simulink model "Motor_realtime"  (R2024a)
settings: Solver=FixedStepAuto  StartTime=0.0  StopTime=10  FixedStep=MotorSampleTime  RelTol=1e-3
model workspace (MAT data in the model file):
  MotorSampleTime = 0.001
undefined symbols (not defined in the file): Serial_Port, Standard_Devices
libraries: sldrtlib x4
settings Model: Creator=17739  LastModifiedBy=17739

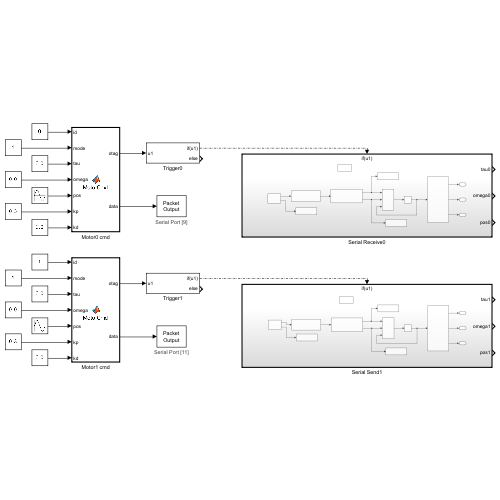
[thumbnail: Simulink's stored preview of the top-level diagram]
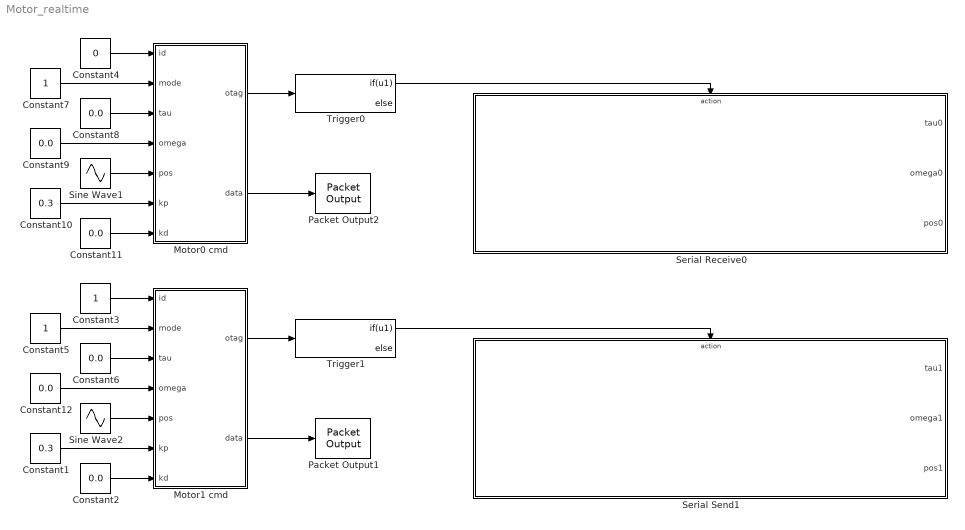
== system Motor_realtime ==
  Constant1 : Constant  Value=0.3
  Constant10 : Constant  Value=0.3
  Constant{2,6,8..9,11..12} (6 alike) : Constant  Value=0.0
  Constant3 : Constant
  Constant4 : Constant  Value=0
  Constant5 : Constant
  Constant7 : Constant
  Motor0 cmd : MATLAB Function  TreatAsAtomicUnit=on
  Motor1 cmd : MATLAB Function  TreatAsAtomicUnit=on
  Packet Output1 : sldrtlib/Packet Output  SampleTime=MotorSampleTime  MaxMissedTicks=inf  ShowMissedTicks=off  YieldWhenWaiting=off  DrvName=Standard_Devices/Serial_Port  DrvAddress=11  DrvOptions=[4000000 8 0 0 0 0 0 0]  PacketSize=17  DataTypes='17*uint8'  ShowReady=off  ShowError=off  PacketID=1  ByteOrder=1  InitialValue=[]  FinalValue=[]
      settings: AttributesFormatString=Serial Port [11]
  Packet Output2 : sldrtlib/Packet Output  SampleTime=MotorSampleTime  MaxMissedTicks=inf  ShowMissedTicks=off  YieldWhenWaiting=off  DrvName=Standard_Devices/Serial_Port  DrvAddress=9  DrvOptions=[4000000 8 0 0 0 0 0 0]  PacketSize=17  DataTypes='17*uint8'  ShowReady=off  ShowError=off  PacketID=1  ByteOrder=1  InitialValue=[]  FinalValue=[]
      settings: AttributesFormatString=Serial Port [9]
  Serial Receive0 : Subsystem  TreatAsAtomicUnit=on
  Serial Send1 : Subsystem  TreatAsAtomicUnit=on
  Sine Wave1 : Sin  Amplitude=pi  Frequency=pi/5  SampleTime=0
  Sine Wave2 : Sin  Amplitude=pi  Frequency=pi/5  SampleTime=0
  Trigger0 : If  IfExpression=u1
  Trigger1 : If  IfExpression=u1
  wires:
  Constant7/1 -> Motor0 cmd/2(mode)
  Constant11/1 -> Motor0 cmd/7(kd)
  Constant4/1 -> Motor0 cmd/1(id)
  Constant8/1 -> Motor0 cmd/3(tau)
  Constant10/1 -> Motor0 cmd/6(kp)
  Constant9/1 -> Motor0 cmd/4(omega)
  Motor0 cmd/2(data) -> Packet Output2/1
  Sine Wave1/1 -> Motor0 cmd/5(pos)
  Sine Wave2/1 -> Motor1 cmd/5(pos)
  Constant3/1 -> Motor1 cmd/1(id)
  Motor1 cmd/2(data) -> Packet Output1/1
  Constant6/1 -> Motor1 cmd/3(tau)
  Constant5/1 -> Motor1 cmd/2(mode)
  Constant1/1 -> Motor1 cmd/6(kp)
  Constant2/1 -> Motor1 cmd/7(kd)
  Constant12/1 -> Motor1 cmd/4(omega)
  Trigger0/1 -> Serial Receive0/Action
  Motor0 cmd/1(otag) -> Trigger0/1
  Trigger1/1 -> Serial Send1/Action
  Motor1 cmd/1(otag) -> Trigger1/1

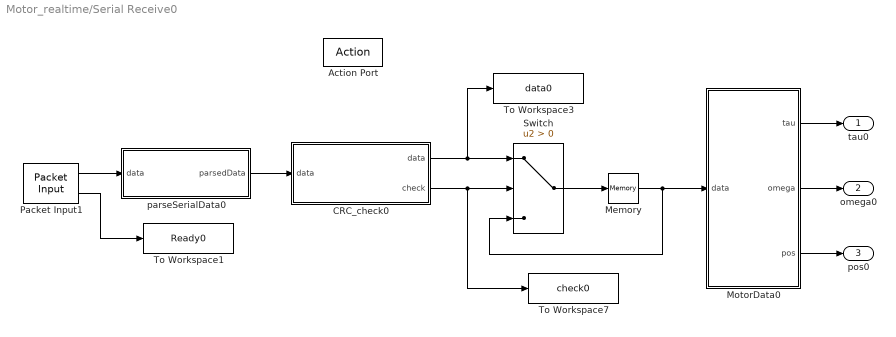
== system Motor_realtime/Serial Receive0 ==
  Action Port : ActionPort  ActionPortLabel=if(u1)
  CRC_check0 : MATLAB Function  TreatAsAtomicUnit=on
  Memory : Memory  InheritSampleTime=on
  MotorData0 : MATLAB Function  TreatAsAtomicUnit=on
  Packet Input1 : sldrtlib/Packet Input  SampleTime=-1  MaxMissedTicks=inf  ShowMissedTicks=off  YieldWhenWaiting=off  DrvName=Standard_Devices/Serial_Port  DrvAddress=9  DrvOptions=[4000000 8 0 0 0 0 0 0]  PacketSize=16  DataTypes='16*uint8'  ShowReady=on  ShowError=off  PacketID=1  ByteOrder=1  ShowTimestamp=off
      settings: AttributesFormatString=Serial Port [9]
  Switch : Switch  Criteria=u2 > Threshold  SaturateOnIntegerOverflow=off  InputSameDT=off
  To Workspace1 : ToWorkspace  VariableName=Ready0  SampleTime=-1
  To Workspace3 : ToWorkspace  VariableName=data0  SampleTime=-1
  To Workspace7 : ToWorkspace  VariableName=check0  SampleTime=-1
  parseSerialData0 : MATLAB Function  TreatAsAtomicUnit=on
  tau0 : Outport
  omega0 : Outport  Port=2
  pos0 : Outport  Port=3
  wires:
  Switch/1 -> Memory/1
  CRC_check0/1(data) -> To Workspace3/1, Switch/1
  CRC_check0/2(check) -> Switch/2, To Workspace7/1
  parseSerialData0/1(parsedData) -> CRC_check0/1("data ")
  Memory/1 -> MotorData0/1(data), Switch/3
  Packet Input1/1 -> parseSerialData0/1(data)
  Packet Input1/2 -> To Workspace1/1
  MotorData0/1(tau) -> tau0/1
  MotorData0/2(omega) -> omega0/1
  MotorData0/3(pos) -> pos0/1

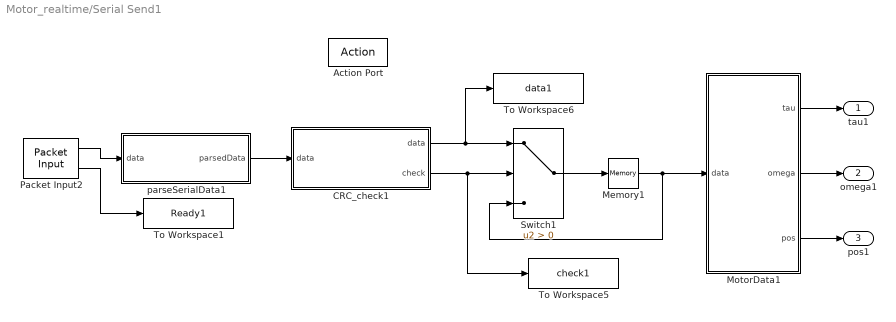
== system Motor_realtime/Serial Send1 ==
  Action Port : ActionPort  ActionPortLabel=if(u1)
  CRC_check1 : MATLAB Function  TreatAsAtomicUnit=on
  Memory1 : Memory  InheritSampleTime=on
  MotorData1 : MATLAB Function  TreatAsAtomicUnit=on
  Packet Input2 : sldrtlib/Packet Input  SampleTime=-1  MaxMissedTicks=inf  ShowMissedTicks=off  YieldWhenWaiting=off  DrvName=Standard_Devices/Serial_Port  DrvAddress=11  DrvOptions=[4000000 8 0 0 0 0 0 0]  PacketSize=16  DataTypes='16*uint8'  ShowReady=on  ShowError=off  PacketID=1  ByteOrder=1  ShowTimestamp=off
      settings: AttributesFormatString=Serial Port [11]
  Switch1 : Switch  Criteria=u2 > Threshold  SaturateOnIntegerOverflow=off  InputSameDT=off
  To Workspace1 : ToWorkspace  VariableName=Ready1  SampleTime=-1
  To Workspace5 : ToWorkspace  VariableName=check1  SampleTime=-1
  To Workspace6 : ToWorkspace  VariableName=data1  SampleTime=-1
  parseSerialData1 : MATLAB Function  TreatAsAtomicUnit=on
  tau1 : Outport
  omega1 : Outport  Port=2
  pos1 : Outport  Port=3
  wires:
  CRC_check1/1(data) -> To Workspace6/1, Switch1/1
  CRC_check1/2(check) -> Switch1/2, To Workspace5/1
  Switch1/1 -> Memory1/1
  Memory1/1 -> MotorData1/1(data), Switch1/3
  parseSerialData1/1(parsedData) -> CRC_check1/1("data ")
  Packet Input2/1 -> parseSerialData1/1(data)
  MotorData1/3(pos) -> pos1/1
  MotorData1/2(omega) -> omega1/1
  MotorData1/1(tau) -> tau1/1
  Packet Input2/2 -> To Workspace1/1

== matlab function Motor_realtime/Serial Send1/parseSerialData1 ==
  data: data input; parsedData output
function parsedData = parseSerialData(data)
    persistent buffer;
    if isempty(buffer)
        buffer = uint8([]);
    end

    % Append new data to buffer, ensuring data is a row vector
    buffer = [buffer, data(:)']; 

    % Define header and data size
    header = uint8([253, 238]); % 定义包头
    dataSize = 16; % 你的数据包大小

    % Initialize parsedData as an empty uint8 array of size 16
    parsedData = uint8([253, 238, zeros(1, dataSize-2)]);

    % Check if the buffer contains a valid packet
    while length(buffer) >= dataSize
        % Find the header in the buffer
        headerPos = findHeader(buffer, header);

        % If header is found and there is enough data for a full packet
        if ~isempty(headerPos) && (headerPos(1) + dataSize - 1 <= length(buffer))
            % Extract the valid packet
            for num = 1:dataSize
                parsedData(num) = buffer(headerPos(1) + num - 1);
            end
            % Remove the extracted packet from the buffer
            if length(headerPos) > 1
                buffer = buffer(headerPos(2):end);
            else
                buffer = buffer((headerPos(1) + dataSize):end);
            end
            return; % Exit the function after finding the first valid packet
        else
            % If no valid packet is found, clear the buffer up to the header position
            if ~isempty(headerPos)
                buffer = buffer(headerPos(1):end);
            else
                buffer = uint8([]);
            end
            break;
        end
    end
end

function pos = findHeader(buffer, header)
    pos = [];
    for i = 1:(length(buffer) - length(header) + 1)
        if all(buffer(i:i + length(header) - 1) == header)
            pos = i;
            return;
        end
    end
end

== matlab function Motor_realtime/Motor0 cmd ==
  data: otag output boolean size=1; data output size=[1 17]; id input; mode input; tau input; omega input; pos input; kp input; kd input
function [otag, data] = MotorCmd(id, mode, tau, omega, pos, kp, kd)
otag = true;
data = uint8([hex2dec('FE'), hex2dec('EE'), ...
    mode*16 + id, ...
    typecast(int16(fix(tau * 256)), 'uint8'), ...
    typecast(int16(fix(omega / (2 * pi) * 256)), 'uint8'), ...
    typecast(int32(fix(pos / (2 * pi) * 32768)), 'uint8'), ...
    typecast(int16(fix(kp * 1280)), 'uint8'), ...
    typecast(int16(fix(kd * 1280)), 'uint8'), ...
    0, 0]); % CRC16 计算稍后添加

% 计算并添加 CRC16 校验
crc = calculateCRC(data(1:15)); % 自定义 CRC 计算函数
data(16:17) = typecast(uint16(crc), 'uint8');
end
% 自定义 CRC 计算函数
function crc = calculateCRC(data)
crc_ccitt_table = [
    0x0000, 0x1189, 0x2312, 0x329b, 0x4624, 0x57ad, 0x6536, 0x74bf, ...
    0x8c48, 0x9dc1, 0xaf5a, 0xbed3, 0xca6c, 0xdbe5, 0xe97e, 0xf8f7, ...
    0x1081, 0x0108, 0x3393, 0x221a, 0x56a5, 0x472c, 0x75b7, 0x643e, ...
    0x9cc9, 0x8d40, 0xbfdb, 0xae52, 0xdaed, 0xcb64, 0xf9ff, 0xe876, ...
    0x2102, 0x308b, 0x0210, 0x1399, 0x6726, 0x76af, 0x4434, 0x55bd, ...
    0xad4a, 0xbcc3, 0x8e58, 0x9fd1, 0xeb6e, 0xfae7, 0xc87c, 0xd9f5, ...
    0x3183, 0x200a, 0x1291, 0x0318, 0x77a7, 0x662e, 0x54b5, 0x453c, ...
    0xbdcb, 0xac42, 0x9ed9, 0x8f50, 0xfbef, 0xea66, 0xd8fd, 0xc974, ...
    0x4204, 0x538d, 0x6116, 0x709f, 0x0420, 0x15a9, 0x2732, 0x36bb, ...
    0xce4c, 0xdfc5, 0xed5e, 0xfcd7, 0x8868, 0x99e1, 0xab7a, 0xbaf3, ...
    0x5285, 0x430c, 0x7197, 0x601e, 0x14a1, 0x0528, 0x37b3, 0x263a, ...
    0xdecd, 0xcf44, 0xfddf, 0xec56, 0x98e9, 0x8960, 0xbbfb, 0xaa72, ...
    0x6306, 0x728f, 0x4014, 0x519d, 0x2522, 0x34ab, 0x0630, 0x17b9, ...
    0xef4e, 0xfec7, 0xcc5c, 0xddd5, 0xa96a, 0xb8e3, 0x8a78, 0x9bf1, ...
    0x7387, 0x620e, 0x5095, 0x411c, 0x35a3, 0x242a, 0x16b1, 0x0738, ...
    0xffcf, 0xee46, 0xdcdd, 0xcd54, 0xb9eb, 0xa862, 0x9af9, 0x8b70, ...
    0x8408, 0x9581, 0xa71a, 0xb693, 0xc22c, 0xd3a5, 0xe13e, 0xf0b7, ...
    0x0840, 0x19c9, 0x2b52, 0x3adb, 0x4e64, 0x5fed, 0x6d76, 0x7cff, ...
    0x9489, 0x8500, 0xb79b, 0xa612, 0xd2ad, 0xc324, 0xf1bf, 0xe036, ...
    0x18c1, 0x0948, 0x3bd3, 0x2a5a, 0x5ee5, 0x4f6c, 0x7df7, 0x6c7e, ...
    0xa50a, 0xb483, 0x8618, 0x9791, 0xe32e, 0xf2a7, 0xc03c, 0xd1b5, ...
    0x2942, 0x38cb, 0x0a50, 0x1bd9, 0x6f66, 0x7eef, 0x4c74, 0x5dfd, ...
    0xb58b, 0xa402, 0x9699, 0x8710, 0xf3af, 0xe226, 0xd0bd, 0xc134, ...
    0x39c3, 0x284a, 0x1ad1, 0x0b58, 0x7fe7, 0x6e6e, 0x5cf5, 0x4d7c, ...
    0xc60c, 0xd785, 0xe51e, 0xf497, 0x8028, 0x91a1, 0xa33a, 0xb2b3, ...
    0x4a44, 0x5bcd, 0x6956, 0x78df, 0x0c60, 0x1de9, 0x2f72, 0x3efb, ...
    0xd68d, 0xc704, 0xf59f, 0xe416, 0x90a9, 0x8120, 0xb3bb, 0xa232, ...
    0x5ac5, 0x4b4c, 0x79d7, 0x685e, 0x1ce1, 0x0d68, 0x3ff3, 0x2e7a, ...
    0xe70e, 0xf687, 0xc41c, 0xd595, 0xa12a, 0xb0a3, 0x8238, 0x93b1, ...
    0x6b46, 0x7acf, 0x4854, 0x59dd, 0x2d62, 0x3ceb, 0x0e70, 0x1ff9, ...
    0xf78f, 0xe606, 0xd49d, 0xc514, 0xb1ab, 0xa022, 0x92b9, 0x8330, ...
    0x7bc7, 0x6a4e, 0x58d5, 0x495c, 0x3de3, 0x2c6a, 0x1ef1, 0x0f78 ...
    ];

crc = uint16(0);
for i = 1:length(data)
    tableIndex = bitand(bitxor(crc, uint16(data(i))), uint16(0xff));
    crc = bitxor(bitshift(crc, -8), crc_ccitt_table(tableIndex + 1));
end
end

== matlab function Motor_realtime/Motor1 cmd ==
  data: otag output size=1; data output size=[1 17]; id input; mode input; tau input; omega input; pos input; kp input; kd input
function [otag, data] = MotorCmd(id, mode, tau, omega, pos, kp, kd)
otag = true;
data = uint8([hex2dec('FE'), hex2dec('EE'), ...
    mode*16 + id, ...
    typecast(int16(fix(tau * 256)), 'uint8'), ...
    typecast(int16(fix(omega / (2 * pi) * 256)), 'uint8'), ...
    typecast(int32(fix(pos / (2 * pi) * 32768)), 'uint8'), ...
    typecast(int16(fix(kp * 1280)), 'uint8'), ...
    typecast(int16(fix(kd * 1280)), 'uint8'), ...
    0, 0]); % CRC16 计算稍后添加

% 计算并添加 CRC16 校验
crc = calculateCRC(data(1:15)); % 自定义 CRC 计算函数
data(16:17) = typecast(uint16(crc), 'uint8');
end
% 自定义 CRC 计算函数
function crc = calculateCRC(data)
crc_ccitt_table = [
    0x0000, 0x1189, 0x2312, 0x329b, 0x4624, 0x57ad, 0x6536, 0x74bf, ...
    0x8c48, 0x9dc1, 0xaf5a, 0xbed3, 0xca6c, 0xdbe5, 0xe97e, 0xf8f7, ...
    0x1081, 0x0108, 0x3393, 0x221a, 0x56a5, 0x472c, 0x75b7, 0x643e, ...
    0x9cc9, 0x8d40, 0xbfdb, 0xae52, 0xdaed, 0xcb64, 0xf9ff, 0xe876, ...
    0x2102, 0x308b, 0x0210, 0x1399, 0x6726, 0x76af, 0x4434, 0x55bd, ...
    0xad4a, 0xbcc3, 0x8e58, 0x9fd1, 0xeb6e, 0xfae7, 0xc87c, 0xd9f5, ...
    0x3183, 0x200a, 0x1291, 0x0318, 0x77a7, 0x662e, 0x54b5, 0x453c, ...
    0xbdcb, 0xac42, 0x9ed9, 0x8f50, 0xfbef, 0xea66, 0xd8fd, 0xc974, ...
    0x4204, 0x538d, 0x6116, 0x709f, 0x0420, 0x15a9, 0x2732, 0x36bb, ...
    0xce4c, 0xdfc5, 0xed5e, 0xfcd7, 0x8868, 0x99e1, 0xab7a, 0xbaf3, ...
    0x5285, 0x430c, 0x7197, 0x601e, 0x14a1, 0x0528, 0x37b3, 0x263a, ...
    0xdecd, 0xcf44, 0xfddf, 0xec56, 0x98e9, 0x8960, 0xbbfb, 0xaa72, ...
    0x6306, 0x728f, 0x4014, 0x519d, 0x2522, 0x34ab, 0x0630, 0x17b9, ...
    0xef4e, 0xfec7, 0xcc5c, 0xddd5, 0xa96a, 0xb8e3, 0x8a78, 0x9bf1, ...
    0x7387, 0x620e, 0x5095, 0x411c, 0x35a3, 0x242a, 0x16b1, 0x0738, ...
    0xffcf, 0xee46, 0xdcdd, 0xcd54, 0xb9eb, 0xa862, 0x9af9, 0x8b70, ...
    0x8408, 0x9581, 0xa71a, 0xb693, 0xc22c, 0xd3a5, 0xe13e, 0xf0b7, ...
    0x0840, 0x19c9, 0x2b52, 0x3adb, 0x4e64, 0x5fed, 0x6d76, 0x7cff, ...
    0x9489, 0x8500, 0xb79b, 0xa612, 0xd2ad, 0xc324, 0xf1bf, 0xe036, ...
    0x18c1, 0x0948, 0x3bd3, 0x2a5a, 0x5ee5, 0x4f6c, 0x7df7, 0x6c7e, ...
    0xa50a, 0xb483, 0x8618, 0x9791, 0xe32e, 0xf2a7, 0xc03c, 0xd1b5, ...
    0x2942, 0x38cb, 0x0a50, 0x1bd9, 0x6f66, 0x7eef, 0x4c74, 0x5dfd, ...
    0xb58b, 0xa402, 0x9699, 0x8710, 0xf3af, 0xe226, 0xd0bd, 0xc134, ...
    0x39c3, 0x284a, 0x1ad1, 0x0b58, 0x7fe7, 0x6e6e, 0x5cf5, 0x4d7c, ...
    0xc60c, 0xd785, 0xe51e, 0xf497, 0x8028, 0x91a1, 0xa33a, 0xb2b3, ...
    0x4a44, 0x5bcd, 0x6956, 0x78df, 0x0c60, 0x1de9, 0x2f72, 0x3efb, ...
    0xd68d, 0xc704, 0xf59f, 0xe416, 0x90a9, 0x8120, 0xb3bb, 0xa232, ...
    0x5ac5, 0x4b4c, 0x79d7, 0x685e, 0x1ce1, 0x0d68, 0x3ff3, 0x2e7a, ...
    0xe70e, 0xf687, 0xc41c, 0xd595, 0xa12a, 0xb0a3, 0x8238, 0x93b1, ...
    0x6b46, 0x7acf, 0x4854, 0x59dd, 0x2d62, 0x3ceb, 0x0e70, 0x1ff9, ...
    0xf78f, 0xe606, 0xd49d, 0xc514, 0xb1ab, 0xa022, 0x92b9, 0x8330, ...
    0x7bc7, 0x6a4e, 0x58d5, 0x495c, 0x3de3, 0x2c6a, 0x1ef1, 0x0f78 ...
    ];

crc = uint16(0);
for i = 1:length(data)
    tableIndex = bitand(bitxor(crc, uint16(data(i))), uint16(0xff));
    crc = bitxor(bitshift(crc, -8), crc_ccitt_table(tableIndex + 1));
end
end

== matlab function Motor_realtime/Serial Send1/CRC_check1 ==
  data: data output; check output; data input
function [data, check] = CRC_Check(data)
crc_ccitt_table = [
    0x0000, 0x1189, 0x2312, 0x329b, 0x4624, 0x57ad, 0x6536, 0x74bf, ...
    0x8c48, 0x9dc1, 0xaf5a, 0xbed3, 0xca6c, 0xdbe5, 0xe97e, 0xf8f7, ...
    0x1081, 0x0108, 0x3393, 0x221a, 0x56a5, 0x472c, 0x75b7, 0x643e, ...
    0x9cc9, 0x8d40, 0xbfdb, 0xae52, 0xdaed, 0xcb64, 0xf9ff, 0xe876, ...
    0x2102, 0x308b, 0x0210, 0x1399, 0x6726, 0x76af, 0x4434, 0x55bd, ...
    0xad4a, 0xbcc3, 0x8e58, 0x9fd1, 0xeb6e, 0xfae7, 0xc87c, 0xd9f5, ...
    0x3183, 0x200a, 0x1291, 0x0318, 0x77a7, 0x662e, 0x54b5, 0x453c, ...
    0xbdcb, 0xac42, 0x9ed9, 0x8f50, 0xfbef, 0xea66, 0xd8fd, 0xc974, ...
    0x4204, 0x538d, 0x6116, 0x709f, 0x0420, 0x15a9, 0x2732, 0x36bb, ...
    0xce4c, 0xdfc5, 0xed5e, 0xfcd7, 0x8868, 0x99e1, 0xab7a, 0xbaf3, ...
    0x5285, 0x430c, 0x7197, 0x601e, 0x14a1, 0x0528, 0x37b3, 0x263a, ...
    0xdecd, 0xcf44, 0xfddf, 0xec56, 0x98e9, 0x8960, 0xbbfb, 0xaa72, ...
    0x6306, 0x728f, 0x4014, 0x519d, 0x2522, 0x34ab, 0x0630, 0x17b9, ...
    0xef4e, 0xfec7, 0xcc5c, 0xddd5, 0xa96a, 0xb8e3, 0x8a78, 0x9bf1, ...
    0x7387, 0x620e, 0x5095, 0x411c, 0x35a3, 0x242a, 0x16b1, 0x0738, ...
    0xffcf, 0xee46, 0xdcdd, 0xcd54, 0xb9eb, 0xa862, 0x9af9, 0x8b70, ...
    0x8408, 0x9581, 0xa71a, 0xb693, 0xc22c, 0xd3a5, 0xe13e, 0xf0b7, ...
    0x0840, 0x19c9, 0x2b52, 0x3adb, 0x4e64, 0x5fed, 0x6d76, 0x7cff, ...
    0x9489, 0x8500, 0xb79b, 0xa612, 0xd2ad, 0xc324, 0xf1bf, 0xe036, ...
    0x18c1, 0x0948, 0x3bd3, 0x2a5a, 0x5ee5, 0x4f6c, 0x7df7, 0x6c7e, ...
    0xa50a, 0xb483, 0x8618, 0x9791, 0xe32e, 0xf2a7, 0xc03c, 0xd1b5, ...
    0x2942, 0x38cb, 0x0a50, 0x1bd9, 0x6f66, 0x7eef, 0x4c74, 0x5dfd, ...
    0xb58b, 0xa402, 0x9699, 0x8710, 0xf3af, 0xe226, 0xd0bd, 0xc134, ...
    0x39c3, 0x284a, 0x1ad1, 0x0b58, 0x7fe7, 0x6e6e, 0x5cf5, 0x4d7c, ...
    0xc60c, 0xd785, 0xe51e, 0xf497, 0x8028, 0x91a1, 0xa33a, 0xb2b3, ...
    0x4a44, 0x5bcd, 0x6956, 0x78df, 0x0c60, 0x1de9, 0x2f72, 0x3efb, ...
    0xd68d, 0xc704, 0xf59f, 0xe416, 0x90a9, 0x8120, 0xb3bb, 0xa232, ...
    0x5ac5, 0x4b4c, 0x79d7, 0x685e, 0x1ce1, 0x0d68, 0x3ff3, 0x2e7a, ...
    0xe70e, 0xf687, 0xc41c, 0xd595, 0xa12a, 0xb0a3, 0x8238, 0x93b1, ...
    0x6b46, 0x7acf, 0x4854, 0x59dd, 0x2d62, 0x3ceb, 0x0e70, 0x1ff9, ...
    0xf78f, 0xe606, 0xd49d, 0xc514, 0xb1ab, 0xa022, 0x92b9, 0x8330, ...
    0x7bc7, 0x6a4e, 0x58d5, 0x495c, 0x3de3, 0x2c6a, 0x1ef1, 0x0f78 ...
    ];

crc = uint16(0);
for i = 1:14
    tableIndex = bitand(bitxor(crc, uint16(data(i))), uint16(0xff));
    crc = bitxor(bitshift(crc, -8), crc_ccitt_table(tableIndex + 1));
end
check = false;
if typecast(uint8(data(end-1:end)), 'uint16') == crc
    check = true;
end
end

== matlab function Motor_realtime/Serial Send1/MotorData1 ==
  data: data input; tau output size=1; omega output size=1; pos output size=1
function [tau, omega, pos] = MotorData(data)
tau = double(typecast(uint8(data(4:5)), 'int16')) / 256;
omega = double(typecast(uint8(data(6:7)), 'int16')) / 256 * 2 * pi;
pos = double(typecast(uint8(data(8:11)), 'int32')) / 32768 * 2 * pi;
end

== matlab function Motor_realtime/Serial Receive0/CRC_check0 ==
  data: data output size=[1 16]; check output; data input
function [data, check] = CRC_Check(data)

crc_ccitt_table = [
    0x0000, 0x1189, 0x2312, 0x329b, 0x4624, 0x57ad, 0x6536, 0x74bf, ...
    0x8c48, 0x9dc1, 0xaf5a, 0xbed3, 0xca6c, 0xdbe5, 0xe97e, 0xf8f7, ...
    0x1081, 0x0108, 0x3393, 0x221a, 0x56a5, 0x472c, 0x75b7, 0x643e, ...
    0x9cc9, 0x8d40, 0xbfdb, 0xae52, 0xdaed, 0xcb64, 0xf9ff, 0xe876, ...
    0x2102, 0x308b, 0x0210, 0x1399, 0x6726, 0x76af, 0x4434, 0x55bd, ...
    0xad4a, 0xbcc3, 0x8e58, 0x9fd1, 0xeb6e, 0xfae7, 0xc87c, 0xd9f5, ...
    0x3183, 0x200a, 0x1291, 0x0318, 0x77a7, 0x662e, 0x54b5, 0x453c, ...
    0xbdcb, 0xac42, 0x9ed9, 0x8f50, 0xfbef, 0xea66, 0xd8fd, 0xc974, ...
    0x4204, 0x538d, 0x6116, 0x709f, 0x0420, 0x15a9, 0x2732, 0x36bb, ...
    0xce4c, 0xdfc5, 0xed5e, 0xfcd7, 0x8868, 0x99e1, 0xab7a, 0xbaf3, ...
    0x5285, 0x430c, 0x7197, 0x601e, 0x14a1, 0x0528, 0x37b3, 0x263a, ...
    0xdecd, 0xcf44, 0xfddf, 0xec56, 0x98e9, 0x8960, 0xbbfb, 0xaa72, ...
    0x6306, 0x728f, 0x4014, 0x519d, 0x2522, 0x34ab, 0x0630, 0x17b9, ...
    0xef4e, 0xfec7, 0xcc5c, 0xddd5, 0xa96a, 0xb8e3, 0x8a78, 0x9bf1, ...
    0x7387, 0x620e, 0x5095, 0x411c, 0x35a3, 0x242a, 0x16b1, 0x0738, ...
    0xffcf, 0xee46, 0xdcdd, 0xcd54, 0xb9eb, 0xa862, 0x9af9, 0x8b70, ...
    0x8408, 0x9581, 0xa71a, 0xb693, 0xc22c, 0xd3a5, 0xe13e, 0xf0b7, ...
    0x0840, 0x19c9, 0x2b52, 0x3adb, 0x4e64, 0x5fed, 0x6d76, 0x7cff, ...
    0x9489, 0x8500, 0xb79b, 0xa612, 0xd2ad, 0xc324, 0xf1bf, 0xe036, ...
    0x18c1, 0x0948, 0x3bd3, 0x2a5a, 0x5ee5, 0x4f6c, 0x7df7, 0x6c7e, ...
    0xa50a, 0xb483, 0x8618, 0x9791, 0xe32e, 0xf2a7, 0xc03c, 0xd1b5, ...
    0x2942, 0x38cb, 0x0a50, 0x1bd9, 0x6f66, 0x7eef, 0x4c74, 0x5dfd, ...
    0xb58b, 0xa402, 0x9699, 0x8710, 0xf3af, 0xe226, 0xd0bd, 0xc134, ...
    0x39c3, 0x284a, 0x1ad1, 0x0b58, 0x7fe7, 0x6e6e, 0x5cf5, 0x4d7c, ...
    0xc60c, 0xd785, 0xe51e, 0xf497, 0x8028, 0x91a1, 0xa33a, 0xb2b3, ...
    0x4a44, 0x5bcd, 0x6956, 0x78df, 0x0c60, 0x1de9, 0x2f72, 0x3efb, ...
    0xd68d, 0xc704, 0xf59f, 0xe416, 0x90a9, 0x8120, 0xb3bb, 0xa232, ...
    0x5ac5, 0x4b4c, 0x79d7, 0x685e, 0x1ce1, 0x0d68, 0x3ff3, 0x2e7a, ...
    0xe70e, 0xf687, 0xc41c, 0xd595, 0xa12a, 0xb0a3, 0x8238, 0x93b1, ...
    0x6b46, 0x7acf, 0x4854, 0x59dd, 0x2d62, 0x3ceb, 0x0e70, 0x1ff9, ...
    0xf78f, 0xe606, 0xd49d, 0xc514, 0xb1ab, 0xa022, 0x92b9, 0x8330, ...
    0x7bc7, 0x6a4e, 0x58d5, 0x495c, 0x3de3, 0x2c6a, 0x1ef1, 0x0f78 ...
    ];

crc = uint16(0);
for i = 1:14
    tableIndex = bitand(bitxor(crc, uint16(data(i))), uint16(0xff));
    crc = bitxor(bitshift(crc, -8), crc_ccitt_table(tableIndex + 1));
end
check = false;
if typecast(uint8(data(end-1:end)), 'uint16') == crc
    check = true;
end
end

== matlab function Motor_realtime/Serial Receive0/MotorData0 ==
  data: data input; tau output size=1; omega output size=1; pos output size=1
function [tau, omega, pos] = MotorData(data)
tau = double(typecast(uint8(data(4:5)), 'int16')) / 256;
omega = double(typecast(uint8(data(6:7)), 'int16')) / 256 * 2 * pi;
pos = double(typecast(uint8(data(8:11)), 'int32')) / 32768 * 2 * pi;
end

== matlab function Motor_realtime/Serial Receive0/parseSerialData0 ==
  data: data input; parsedData output
function parsedData = parseSerialData(data)
    persistent buffer;
    if isempty(buffer)
        buffer = uint8([]);
    end

    % Append new data to buffer, ensuring data is a row vector
    buffer = [buffer, data(:)']; 

    % Define header and data size
    header = uint8([253, 238]); % 定义包头
    dataSize = 16; % 你的数据包大小

    % Initialize parsedData as an empty uint8 array of size 16
    parsedData = uint8([253, 238, zeros(1, dataSize-2)]);

    % Check if the buffer contains a valid packet
    while length(buffer) >= dataSize
        % Find the header in the buffer
        headerPos = findHeader(buffer, header);

        % If header is found and there is enough data for a full packet
        if ~isempty(headerPos) && (headerPos(1) + dataSize - 1 <= length(buffer))
            % Extract the valid packet
            for num = 1:dataSize
                parsedData(num) = buffer(headerPos(1) + num - 1);
            end
            % Remove the extracted packet from the buffer
            if length(headerPos) > 1
                buffer = buffer(headerPos(2):end);
            else
                buffer = buffer((headerPos(1) + dataSize):end);
            end
            return; % Exit the function after finding the first valid packet
        else
            % If no valid packet is found, clear the buffer up to the header position
            if ~isempty(headerPos)
                buffer = buffer(headerPos(1):end);
            else
                buffer = uint8([]);
            end
            break;
        end
    end
end

function pos = findHeader(buffer, header)
    pos = [];
    for i = 1:(length(buffer) - length(header) + 1)
        if all(buffer(i:i + length(header) - 1) == header)
            pos = i;
            return;
        end
    end
end
